simulink model "Target_Control_System"  (R2021b)
settings: Solver=FixedStepDiscrete  StartTime=0.0  StopTime=5  RelTol=1e-3
PreLoadFcn:
  | RTWConfigurationCB('preloadfcn', bdroot);
PostLoadFcn:
  | load('configuration/data_struct.mat');
  | load('configuration/fluxMaps_propMotor.mat');
  | load('configuration/parameterInit_PROP.mat');
  | load('configuration/parameterInit_PUMP.mat');
  | load('configuration/parameterInit_PITCH.mat');
  | load('configuration/parameterInit_TILT.mat');
  | %load('configuration/base_workspace_signal_definition.mat');
  | %load('resolvedatastores_to_baseworkspace_for_faster_simulation.mat');
model workspace (MAT data in the model file):
  SIMULATION_OPTIONS : Simulink.Parameter (value not decoded)
  TARGET_CODE_GEN : Simulink.Parameter (value not decoded)
  TCS_SAMPLE_FREQ_HZ : Simulink.Parameter (value not decoded)
symbols that are objects in the model workspace (value not decoded): TARGET_CODE_GEN, TCS_SAMPLE_FREQ_HZ
undefined symbols (not defined in the file): A_DQ_REF_LPF_INIT__PITCH, A_DQ_REF_LPF_INIT__PROP, A_DQ_REF_LPF_INIT__PUMP, A_DQ_REF_LPF_INIT__TILT, A_OBSERVER_CONFIDENCE_INIT__PITCH, A_OBSERVER_CONFIDENCE_INIT__PROP, A_OBSERVER_CONFIDENCE_INIT__PUMP, A_OBSERVER_CONFIDENCE_INIT__TILT, ACTUATOR_MAX_ANGLE_TRIP__PITCH, ACTUATOR_MIN_ANGLE_TRIP__PITCH, ACTUATOR_POS_SENSOR_INV_DIRECTION__PITCH, ACTUATOR_POS_SENSOR_INV_DIRECTION__TILT, ACTUATOR_POS_SENSOR_OFFSET__PITCH, ACTUATOR_POS_SENSOR_OFFSET__TILT, ADC_scaler1_baseaddr_TILT, ADC_SCALER_FLOAT_TO_FIXPOINT_EXPANSION, ANGLE_ELEC_FROM_SENSOR_OFFSET_INIT__PITCH, ANGLE_ELEC_FROM_SENSOR_OFFSET_INIT__PROP, ANGLE_ELEC_FROM_SENSOR_OFFSET_INIT__PUMP, ANGLE_ELEC_FROM_SENSOR_OFFSET_INIT__TILT, AUTO_CLEAR_FAULTS_ENABLED__PITCH, AUTO_CLEAR_FAULTS_ENABLED__PROP, AUTO_CLEAR_FAULTS_ENABLED__PUMP, AUTO_CLEAR_FAULTS_ENABLED__TILT, AUTO_CLEAR_FAULTS_WAIT_TICKS__PITCH, AUTO_CLEAR_FAULTS_WAIT_TICKS__PROP, AUTO_CLEAR_FAULTS_WAIT_TICKS__PUMP, AUTO_CLEAR_FAULTS_WAIT_TICKS__TILT, AUTO_I_ZERO_IDLE_TICKS__PITCH, AUTO_I_ZERO_IDLE_TICKS__PROP, AUTO_I_ZERO_IDLE_TICKS__PUMP, AUTO_I_ZERO_IDLE_TICKS__TILT, AUTO_I_ZERO_OFFSET_IDC_THRESHOLD__PITCH, AUTO_I_ZERO_OFFSET_IDC_THRESHOLD__PROP, AUTO_I_ZERO_OFFSET_IDC_THRESHOLD__PUMP, AUTO_I_ZERO_OFFSET_IDC_THRESHOLD__TILT, AUTO_I_ZERO_OFFSET_IPH_THRESHOLD__PITCH, AUTO_I_ZERO_OFFSET_IPH_THRESHOLD__PROP, AUTO_I_ZERO_OFFSET_IPH_THRESHOLD__PUMP, AUTO_I_ZERO_OFFSET_IPH_THRESHOLD__TILT, AUTO_SENSORLESS_SWITCHOVER_DISABLE_OMEGA, AUTO_SENSORLESS_SWITCHOVER_ENABLE_OMEGA, AUTO_SENSORLESS_SWITCHOVER_MIN_CONFIDENCE, AUXILIARY_PROTECTION_UNIT_BASEADDR__TILT, blanking_max_error_omega_INIT_PITCH, blanking_max_error_omega_INIT_TILT, blanking_max_error_position_INIT_PITCH, blanking_max_error_position_INIT_TILT, BRUTE_START_I_Q_REF_RAMP_SPEED__PITCH, BRUTE_START_I_Q_REF_RAMP_SPEED__PROP, BRUTE_START_I_Q_REF_RAMP_SPEED__PUMP, BRUTE_START_I_Q_REF_RAMP_SPEED__TILT, CONTROL_LOOP_DT_INIT__PITCH, CONTROL_LOOP_DT_INIT__PROP, CONTROL_LOOP_DT_INIT__PUMP, CONTROL_LOOP_DT_INIT__TILT, CORRECTION_FILTER_SCALE__PITCH, CORRECTION_FILTER_SCALE__PROP, CORRECTION_FILTER_SCALE__PUMP, CORRECTION_FILTER_SCALE__TILT ... (+458)
libraries: simulink x178, Reusables_Lib x24
(part 28 of 47)

== system Target_Control_System/Target_Control_System/MainLoop/pitchMotor_mainLoop/mainTask_pitch/motorTaskMainFastStep()/Lowpass Filtered Quantities for External World - Pitch ==
  lpfQuantities : TriggerPort  TriggerType=function-call  VariantControl=Variant
  Constant2 : Constant  Value=0.00008  OutDataTypeStr=single  SampleTime=-1
  Data Store Read27 : DataStoreRead  DataStoreName=oPitch  DataStoreElements=oPitch.oMot_.oParam_.fSlowPassFactor_  IndexOptions=Index vector (dialog)  Indices=1  OutputSizes=1
  Data Store Read28 : DataStoreRead  DataStoreName=oPitch  DataStoreElements=oPitch.oMot_.oIn_.fIPhaseMagnitude_  IndexOptions=Index vector (dialog)  Indices=1  OutputSizes=1
  Data Store Read29 : DataStoreRead  DataStoreName=oPitch  DataStoreElements=oPitch.oMot_.oState_.fIPhaseMagnitudeLpf_  IndexOptions=Index vector (dialog)  Indices=1  OutputSizes=1
  Data Store Read37 : DataStoreRead  DataStoreName=oPitch  DataStoreElements=oPitch.oMot_.oIn_.fId_  IndexOptions=Index vector (dialog)  Indices=1  OutputSizes=1
  Data Store Read42 : DataStoreRead  DataStoreName=oPitch  DataStoreElements=oPitch.oMot_.oIn_.fIq_  IndexOptions=Index vector (dialog)  Indices=1  OutputSizes=1
  Data Store Read43 : DataStoreRead  DataStoreName=oPitch  DataStoreElements=oPitch.oMot_.oOut_.fIdLpf_  IndexOptions=Index vector (dialog)  Indices=1  OutputSizes=1
  Data Store Read44 : DataStoreRead  DataStoreName=oPitch  DataStoreElements=oPitch.oMot_.oOut_.fIqLpf_  IndexOptions=Index vector (dialog)  Indices=1  OutputSizes=1
  Data Store Read46 : DataStoreRead  DataStoreName=oPitch  DataStoreElements=oPitch.oMot_.oOut_.fUdcLpf_  IndexOptions=Index vector (dialog)  Indices=1  OutputSizes=1
  Data Store Read47 : DataStoreRead  DataStoreName=oPitch  DataStoreElements=oPitch.oMot_.oIn_.oAdcData_.fIdc_  IndexOptions=Index vector (dialog)  Indices=1  OutputSizes=1
  Data Store Read48 : DataStoreRead  DataStoreName=oPitch  DataStoreElements=oPitch.oMot_.oOut_.fIdcLpf_  IndexOptions=Index vector (dialog)  Indices=1  OutputSizes=1
  Data Store Read49 : DataStoreRead  DataStoreName=oPitch  DataStoreElements=oPitch.oMot_.oIn_.fPowerDc_  IndexOptions=Index vector (dialog)  Indices=1  OutputSizes=1
  Data Store Read50 : DataStoreRead  DataStoreName=oPitch  DataStoreElements=oPitch.oMot_.oOut_.fPowerDcLpf_  IndexOptions=Index vector (dialog)  Indices=1  OutputSizes=1
  Data Store Read51 : DataStoreRead  DataStoreName=oPitch  DataStoreElements=oPitch.oMot_.oIn_.fTEstimate_  IndexOptions=Index vector (dialog)  Indices=1  OutputSizes=1
  Data Store Read52 : DataStoreRead  DataStoreName=oPitch  DataStoreElements=oPitch.oMot_.oOut_.fTEstimateLpf_  IndexOptions=Index vector (dialog)  Indices=1  OutputSizes=1
  Data Store Read53 : DataStoreRead  DataStoreName=oPitch  DataStoreElements=oPitch.oMot_.oState_.oRampDataIqRef_.fRampOut_  IndexOptions=Index vector (dialog)  Indices=1  OutputSizes=1
  Data Store Read54 : DataStoreRead  DataStoreName=oPitch  DataStoreElements=oPitch.oMot_.oOut_.fIqRefRampOutLpf_  IndexOptions=Index vector (dialog)  Indices=1  OutputSizes=1
  Data Store Read55 : DataStoreRead  DataStoreName=oPitch  DataStoreElements=oPitch.oMot_.oParam_.fADqRefLpf_  IndexOptions=Index vector (dialog)  Indices=1  OutputSizes=1
  Data Store Read56 : DataStoreRead  DataStoreName=oPitch  DataStoreElements=oPitch.oMot_.oIn_.fIdRefTotal_  IndexOptions=Index vector (dialog)  Indices=1  OutputSizes=1
  Data Store Read57 : DataStoreRead  DataStoreName=oPitch  DataStoreElements=oPitch.oMot_.oOut_.fIdRefLpf_  IndexOptions=Index vector (dialog)  Indices=1  OutputSizes=1
  Data Store Read58 : DataStoreRead  DataStoreName=oPitch  DataStoreElements=oPitch.oMot_.oIn_.fUqRef_  IndexOptions=Index vector (dialog)  Indices=1  OutputSizes=1
  Data Store Read59 : DataStoreRead  DataStoreName=oPitch  DataStoreElements=oPitch.oMot_.oOut_.fUqRefLpf_  IndexOptions=Index vector (dialog)  Indices=1  OutputSizes=1
  Data Store Read60 : DataStoreRead  DataStoreName=oPitch  DataStoreElements=oPitch.oMot_.oIn_.fUdRef_  IndexOptions=Index vector (dialog)  Indices=1  OutputSizes=1
  Data Store Read62 : DataStoreRead  DataStoreName=oPitch  DataStoreElements=oPitch.oMot_.oOut_.fUdRefLpf_  IndexOptions=Index vector (dialog)  Indices=1  OutputSizes=1
  Data Store Read63 : DataStoreRead  DataStoreName=oPitch  DataStoreElements=oPitch.oMot_.oOut_.fPowerDcLpf_  IndexOptions=Index vector (dialog)  Indices=1  OutputSizes=1
  Data Store Read64 : DataStoreRead  DataStoreName=oPitch  DataStoreElements=oPitch.oMot_.oOut_.fPowerDcXlpf_  IndexOptions=Index vector (dialog)  Indices=1  OutputSizes=1
  Data Store Read65 : DataStoreRead  DataStoreName=oPitch  DataStoreElements=oPitch.oMot_.oIn_.fOmegaEObserverLpf2_  IndexOptions=Index vector (dialog)  Indices=1  OutputSizes=1
  Data Store Read66 : DataStoreRead  DataStoreName=oPitch  DataStoreElements=oPitch.oMot_.oOut_.fOmegaEObserverXlpf2_  IndexOptions=Index vector (dialog)  Indices=1  OutputSizes=1
  Data Store Read69 : DataStoreRead  DataStoreName=oPitch  DataStoreElements=oPitch.oMot_.oParam_.fAOmegaXfilter2_  IndexOptions=Index vector (dialog)  Indices=1  OutputSizes=1
  Data Store Read77 : DataStoreRead  DataStoreName=oPitch  DataStoreElements=oPitch.oMot_.oIn_.oAdcData_.fUdc_  IndexOptions=Index vector (dialog)  Indices=1  OutputSizes=1
  Data Store Write20 : DataStoreWrite  DataStoreName=oPitch  DataStoreElements=oPitch.oMot_.oState_.fIPhaseMagnitudeLpf_  IndexOptions=Index vector (dialog)  Indices=1  OutputSizes=1
  Data Store Write21 : DataStoreWrite  DataStoreName=oPitch  DataStoreElements=oPitch.oMot_.oOut_.fIdLpf_  IndexOptions=Index vector (dialog)  Indices=1  OutputSizes=1
  Data Store Write22 : DataStoreWrite  DataStoreName=oPitch  DataStoreElements=oPitch.oMot_.oOut_.fIqLpf_  IndexOptions=Index vector (dialog)  Indices=1  OutputSizes=1
  Data Store Write24 : DataStoreWrite  DataStoreName=oPitch  DataStoreElements=oPitch.oMot_.oOut_.fUdcLpf_  IndexOptions=Index vector (dialog)  Indices=1  OutputSizes=1
  Data Store Write25 : DataStoreWrite  DataStoreName=oPitch  DataStoreElements=oPitch.oMot_.oOut_.fIdcLpf_  IndexOptions=Index vector (dialog)  Indices=1  OutputSizes=1
  Data Store Write28 : DataStoreWrite  DataStoreName=oPitch  DataStoreElements=oPitch.oMot_.oOut_.fPowerDcLpf_  IndexOptions=Index vector (dialog)  Indices=1  OutputSizes=1
  Data Store Write29 : DataStoreWrite  DataStoreName=oPitch  DataStoreElements=oPitch.oMot_.oOut_.fTEstimateLpf_  IndexOptions=Index vector (dialog)  Indices=1  OutputSizes=1
  Data Store Write30 : DataStoreWrite  DataStoreName=oPitch  DataStoreElements=oPitch.oMot_.oOut_.fIqRefRampOutLpf_  IndexOptions=Index vector (dialog)  Indices=1  OutputSizes=1
  Data Store Write31 : DataStoreWrite  DataStoreName=oPitch  DataStoreElements=oPitch.oMot_.oOut_.fIdRefLpf_  IndexOptions=Index vector (dialog)  Indices=1  OutputSizes=1
  Data Store Write32 : DataStoreWrite  DataStoreName=oPitch  DataStoreElements=oPitch.oMot_.oOut_.fUqRefLpf_  IndexOptions=Index vector (dialog)  Indices=1  OutputSizes=1
  Data Store Write34 : DataStoreWrite  DataStoreName=oPitch  DataStoreElements=oPitch.oMot_.oOut_.fUdRefLpf_  IndexOptions=Index vector (dialog)  Indices=1  OutputSizes=1
  Data Store Write35 : DataStoreWrite  DataStoreName=oPitch  DataStoreElements=oPitch.oMot_.oOut_.fPowerDcXlpf_  IndexOptions=Index vector (dialog)  Indices=1  OutputSizes=1
  Data Store Write36 : DataStoreWrite  DataStoreName=oPitch  DataStoreElements=oPitch.oMot_.oOut_.fOmegaEObserverXlpf2_  IndexOptions=Index vector (dialog)  Indices=1  OutputSizes=1
  Divide{8..20} (13 alike) : Product  Inputs=**
  Sum{4..5,7,10..11,13,15,18,20..22,25,29} (13 alike) : Sum  Inputs=|+-
  Sum{3,6,8..9,12,14,16..17,19,24,26,30..31} (13 alike) : Sum  Inputs=|++
  wires:
  Data Store Read27/1 -> Divide8/1, Divide9/1, Divide10/1, Divide12/1, Divide13/1, Divide14/1, Divide11/1
  Constant2/1 -> Divide20/1
  Sum12/1 -> Data Store Write25/1
  Sum6/1 -> Data Store Write21/1
  Sum8/1 -> Data Store Write22/1
  Data Store Read49/1 -> Sum11/1
  Data Store Read29/1 -> Sum7/2, Sum3/2
  Sum24/1 -> Data Store Write35/1
  Data Store Read47/1 -> Sum10/1
  Divide17/1 -> Sum30/1
  Sum3/1 -> Data Store Write20/1
  Data Store Read64/1 -> Sum24/2, Sum21/2
  Data Store Read54/1 -> Sum18/2, Sum17/2
  Divide13/1 -> Sum12/1
  Divide11/1 -> Sum14/1
  Divide16/1 -> Sum19/1
  Sum22/1 -> Divide18/2
  Sum15/1 -> Divide14/2
  Sum29/1 -> Divide17/2
  Sum4/1 -> Divide9/2
  Data Store Read58/1 -> Sum29/1
  Divide18/1 -> Sum26/1
  Sum21/1 -> Divide20/2
  Data Store Read42/1 -> Sum5/1
  Data Store Read77/1 -> Sum13/1
  Data Store Read59/1 -> Sum29/2, Sum30/2
  Divide20/1 -> Sum24/1
  Data Store Read69/1 -> Divide18/1
  Sum5/1 -> Divide10/2
  Sum31/1 -> Data Store Write34/1
  Sum16/1 -> Data Store Write29/1
  Sum19/1 -> Data Store Write31/1
  Sum7/1 -> Divide8/2
  Divide10/1 -> Sum8/1
  Data Store Read56/1 -> Sum20/1
  Sum18/1 -> Divide15/2
  Data Store Read28/1 -> Sum7/1
  Sum26/1 -> Data Store Write36/1
  Sum13/1 -> Divide12/2
  Data Store Read55/1 -> Divide15/1, Divide16/1, Divide19/1, Divide17/1
  Data Store Read57/1 -> Sum20/2, Sum19/2
  Divide8/1 -> Sum3/1
  Data Store Read65/1 -> Sum22/1
  Divide9/1 -> Sum6/1
  Data Store Read48/1 -> Sum12/2, Sum10/2
  Divide15/1 -> Sum17/1
  Data Store Read63/1 -> Sum21/1
  Divide14/1 -> Sum16/1
  Data Store Read43/1 -> Sum4/2, Sum6/2
  Data Store Read66/1 -> Sum26/2, Sum22/2
  Data Store Read53/1 -> Sum18/1
  Data Store Read44/1 -> Sum5/2, Sum8/2
  Data Store Read50/1 -> Sum14/2, Sum11/2
  Data Store Read52/1 -> Sum16/2, Sum15/2
  Sum30/1 -> Data Store Write32/1
  Sum17/1 -> Data Store Write30/1
  Data Store Read46/1 -> Sum9/2, Sum13/2
  Data Store Read37/1 -> Sum4/1
  Sum11/1 -> Divide11/2
  Divide12/1 -> Sum9/1
  Data Store Read60/1 -> Sum25/1
  Sum10/1 -> Divide13/2
  Divide19/1 -> Sum31/1
  Sum25/1 -> Divide19/2
  Data Store Read62/1 -> Sum25/2, Sum31/2
  Data Store Read51/1 -> Sum15/1
  Sum14/1 -> Data Store Write28/1
  Sum9/1 -> Data Store Write24/1
  Sum20/1 -> Divide16/2

== system Target_Control_System/Target_Control_System/MainLoop/pitchMotor_mainLoop/mainTask_pitch/motorTaskMainFastStep()/Mechanical System - Pitch ==
  mechanicalSystem : TriggerPort  TriggerType=function-call  VariantControl=Variant
  Data Store Read : DataStoreRead  DataStoreName=oPitch  DataStoreElements=oPitch.oMot_.oState_.oPosSensor_.eInputPositionSensorType_  IndexOptions=Index vector (dialog)  Indices=1  OutputSizes=1
  Enumerated Constant1 : simulink/Sources/Enumerated Constant  OutDataTypeStr=Enum: EPositionSensor_t  Value=EPositionSensor_t.eNone  SampleTime=-1
  NotEqual : RelationalOperator  Operator=~=  OutDataTypeStr=boolean  RndMeth=Simplest
  processSensors(&oPitch) : Subsystem  TreatAsAtomicUnit=on
  wires:
  Enumerated Constant1/1 -> NotEqual/2
  NotEqual/1 -> processSensors(&oPitch)/Enable
  Data Store Read/1 -> NotEqual/1

== system Target_Control_System/Target_Control_System/MainLoop/pitchMotor_mainLoop/mainTask_pitch/motorTaskMainFastStep()/Motor Acceleration - Pitch ==
  note: // Compute the acceleration (derivative of the speed). It is computed simply from the 1-step difference,
      |    // but strongly low pass filtered to ultimately end up with a bandwidth less than 50-100 Hz.
      |    // A filter running at the typical control frequency (80 kHz for the prop) would have to be too steep, so
      |    // a multi-stage, dual sample rate approach is used: A first filter runs at full control rate, with a cut-
      |    // off frequency of some 1-2 kHz. A second filter runs at 5 kHz and brings the bandwidth down to less than
      |    // 50-100 Hz.
      |    // At this location in the code, the first filter stage is executed:
  motorAcceleration : TriggerPort  TriggerType=function-call  VariantControl=Variant
  First filter stage : Subsystem  TreatAsAtomicUnit=on
  Function-Call Generator : simulink/Ports & Subsystems/Function-Call Generator  sample_time=-1  numberOfIterations=1  DisallowWideOutput=off
  Function-Call Split10 : FunctionCallSplit  NumOutputPorts=2
  Speed step : Subsystem
  wires:
  Function-Call Generator/1 -> Function-Call Split10/1
  Function-Call Split10/1 -> First filter stage/Trigger
  Function-Call Split10/2 -> Speed step/Trigger

== system Target_Control_System/Target_Control_System/MainLoop/pitchMotor_mainLoop/mainTask_pitch/motorTaskMainFastStep()/Observer Confidence - Pitch ==
  note: // ideally zero,
      | // but can go up to inf
  note: // Three contributions, each adding 1/3 to give a value in range 0.0-1.0:
      | //  1. Magnitude of estimated flux relative to nominal flux (perhaps not for induction motors)
      | //  REMOVED (for the time being) 2. The relative noise on the magnitude of the estimated flux (relative noise=magnitude of derivative/HPF divided by average value)
      | //  3. The relative noise on the estimated speed
  note: // If greater than 125% off,
      | // keep at 125%
  note: // the 0.4 is 0.5/tempf_max
  note: // 1. magnitude of flux. Map to a 0-0.33 range
  note: // 3. noise on estimated omega
  note: // ideally zero,
      | // but can go up to inf
  note: // If greater than X% off,
      | // keep at X%
  observerConfidence : TriggerPort  TriggerType=function-call  VariantControl=Variant
  Abs2 : Abs  OutDataTypeStr=single
  Abs3 : Abs  OutDataTypeStr=single
  Abs5 : Abs  OutDataTypeStr=single
  Add10 : Sum  Inputs=|-+
  Add11 : Sum
  Add2 : Sum  Inputs=+-
  Add7 : Sum  Inputs=|+-
  Add8 : Sum  Inputs=|-+
  Add9 : Sum  Inputs=|-+
  Automatic switching to sensorless : Subsystem  TreatAsAtomicUnit=on
  Constant14 : Constant  OutDataTypeStr=single  SampleTime=-1
  Data Store Read1 : DataStoreRead  DataStoreName=oPitch  DataStoreElements=oPitch.oMot_.oParam_.fAObserverConfidence_  IndexOptions=Index vector (dialog)  Indices=1  OutputSizes=1
  Data Store Read11 : DataStoreRead  DataStoreName=oPitch  DataStoreElements=oPitch.oMot_.oOut_.fOmegaEObserverXlpf2_  IndexOptions=Index vector (dialog)  Indices=1  OutputSizes=1
  Data Store Read13 : DataStoreRead  DataStoreName=oPitch  DataStoreElements=oPitch.oMot_.oIn_.fFluxMainMagnitudeLpf_  IndexOptions=Index vector (dialog)  Indices=1  OutputSizes=1
  Data Store Read4 : DataStoreRead  DataStoreName=oPitch  DataStoreElements=oPitch.oMot_.oParam_.uiSensorlessSwitchoverMode_  IndexOptions=Index vector (dialog)  Indices=1  OutputSizes=1
  Data Store Read61 : DataStoreRead  DataStoreName=oPitch  DataStoreElements=oPitch.oIsr_.oState_.fOmegaEObserverRaw2_  IndexOptions=Index vector (dialog)  Indices=1  OutputSizes=1
  Data Store Read83 : DataStoreRead  DataStoreName=oPitch  DataStoreElements=oPitch.oMot_.oParam_.fMainFluxNominal_  IndexOptions=Index vector (dialog)  Indices=1  OutputSizes=1
  Data Store Write33 : DataStoreWrite  DataStoreName=oPitch  DataStoreElements=oPitch.oMot_.oState_.fObserverConfidence_  IndexOptions=Index vector (dialog)  Indices=1  OutputSizes=1
  Divide1 : Product  Inputs=*/
  Divide3 : Product  Inputs=*/
  Gain11 : Gain  Gain=0.83
  Gain5 : Gain  Gain=0.4
  Half : Constant  Value=0.5  OutDataTypeStr=single  SampleTime=-1
  Half2 : Constant  Value=0.5  OutDataTypeStr=single  SampleTime=-1
  IIR : Subsystem
  Saturation2 : Saturate  UpperLimit=1.25  LowerLimit=-inf
  Saturation3 : Saturate  UpperLimit=0.6  LowerLimit=-inf
  Switch3 : Switch  Criteria=u2 > Threshold  Threshold=0.5
  Zero8 : Constant  Value=0  OutDataTypeStr=Inherit: Inherit via back propagation  SampleTime=-1
  isNaN : RelationalOperator  Operator=isNaN  OutDataTypeStr=boolean  RndMeth=Simplest
  wires:
  Zero8/1 -> Switch3/1
  Half2/1 -> Add10/2
  Data Store Read13/1 -> Add7/1
  Data Store Read4/1 -> Automatic switching to sensorless/Enable
  Half/1 -> Add8/2
  Switch3/1 -> IIR/1(In)  "fObserverConfidenceRaw"
  Divide3/1 -> Saturation3/1
  Data Store Read83/1 -> Add7/2, Divide1/2
  Data Store Read11/1 -> Abs5/1, Add9/2
  Add10/1 -> Add11/2
  Abs5/1 -> Divide3/2
  Constant14/1 -> Add2/1
  Add8/1 -> Add11/1
  Data Store Read1/1 -> IIR/3(K), Add2/2
  Saturation2/1 -> Gain5/1  "fTemp"
  Divide1/1 -> Saturation2/1
  Add7/1 -> Abs2/1
  Gain11/1 -> Add10/1
  IIR/1(Out) -> Automatic switching to sensorless/1(In1), Data Store Write33/1
  Add11/1 -> Switch3/3, isNaN/1  "fObserverConfidenceRaw"
  Add9/1 -> Abs3/1
  Add2/1 -> IIR/2(1-K)
  Abs3/1 -> Divide3/1
  Abs2/1 -> Divide1/1
  isNaN/1 -> Switch3/2
  Saturation3/1 -> Gain11/1
  Data Store Read61/1 -> Add9/1
  Gain5/1 -> Add8/1

== system Target_Control_System/Target_Control_System/MainLoop/pitchMotor_mainLoop/mainTask_pitch/motorTaskMainFastStep()/Software Overcurrent Protection - Pitch ==
  overcurrentProtection : TriggerPort  TriggerType=function-call  VariantControl=Variant
  Constant7 : Constant  Value=211  OutDataTypeStr=uint32  SampleTime=-1
  Constant8 : Constant  Value=212  OutDataTypeStr=uint32  SampleTime=-1
  Data Store Read45 : DataStoreRead  DataStoreName=oPitch  DataStoreElements=oPitch.oMot_.oIn_.fIPhaseMagnitude_  IndexOptions=Index vector (dialog)  Indices=1  OutputSizes=1
  Data Store Read79 : DataStoreRead  DataStoreName=oPitch  DataStoreElements=oPitch.oMot_.oState_.uiDriveState_  IndexOptions=Index vector (dialog)  Indices=1  OutputSizes=1
  Data Store Read81 : DataStoreRead  DataStoreName=oPitch  DataStoreElements=oPitch.oMot_.oParam_.fTripLimitSoftwareA_  IndexOptions=Index vector (dialog)  Indices=1  OutputSizes=1
  Equal1 : RelationalOperator  Operator===  OutDataTypeStr=boolean  RndMeth=Simplest
  Equal2 : RelationalOperator  Operator===  OutDataTypeStr=boolean  RndMeth=Simplest
  Forced_angle_overcurrent : Subsystem  TreatAsAtomicUnit=on
  GreaterThan3 : RelationalOperator  Operator=>  OutDataTypeStr=boolean  RndMeth=Simplest
  OR : Logic  Operator=OR  AllPortsSameDT=off  OutDataTypeStr=boolean
  checkForHwOvercurrents(&oPitch) : Subsystem  TreatAsAtomicUnit=on
  softwareOvercurrentProtection : Stateflow chart  TreatAsAtomicUnit=on
  wires:
  Constant8/1 -> Equal2/1
  Equal2/1 -> OR/1
  Equal1/1 -> OR/2
  OR/1 -> Forced_angle_overcurrent/Enable
  Data Store Read79/1 -> Equal1/1, Equal2/2
  Constant7/1 -> Equal1/2
  GreaterThan3/1 -> checkForHwOvercurrents(&oPitch)/Enable
  Data Store Read45/1 -> GreaterThan3/1
  Data Store Read81/1 -> GreaterThan3/2

== system Target_Control_System/Target_Control_System/MainLoop/propMotor_mainLoop/Decimation gate A for 200 Hz Prop/Current offset nulling/initiateOffsetNulling(&oProp) ==
  note: Further checks for starting the nulling process are handled inside the lower level function
  Enable : EnablePort
  Chart : Stateflow chart  TreatAsAtomicUnit=on

== system Target_Control_System/Target_Control_System/MainLoop/propMotor_mainLoop/Decimation gate A for 200 Hz Prop/Subsystem/Subsystem ==
  Enable : EnablePort
  Data Store Write1 : DataStoreWrite  DataStoreName=oProp  DataStoreElements=oProp.oMot_.oState_.fIdleCtrlCurrent_  IndexOptions=Index vector (dialog)  Indices=1  OutputSizes=1
  Data Store Write3 : DataStoreWrite  DataStoreName=oProp  DataStoreElements=oProp.oMot_.oParam_.oPiDataIdleCtrl_.fState_  IndexOptions=Index vector (dialog)  Indices=1  OutputSizes=1
  Zero1 : Constant  Value=0  OutDataTypeStr=single  SampleTime=-1
  wires:
  Zero1/1 -> Data Store Write1/1, Data Store Write3/1

== system Target_Control_System/Target_Control_System/MainLoop/propMotor_mainLoop/Decimation gate A for 200 Hz Prop/Subsystem/piControllerStep_Idle_Controller ==
  fActual : Inport
  fTarget : Inport  Port=2
  fKp : Inport  Port=3
  fKi : Inport  Port=4
  fScale : Inport  Port=5
  fLoopDt : Inport  Port=6
  fIntMax : Inport  Port=7
  fOutMax : Inport  Port=8
  fIntMin : Inport  Port=9
  fOutMin : Inport  Port=10
  fState : Inport  Port=11
  Enable : EnablePort
  Add : Sum  Inputs=|++
  Data Store Write11 : DataStoreWrite  DataStoreName=oProp  DataStoreElements=oProp.oMot_.oState_.fIdleCtrlCurrent_  IndexOptions=Index vector (dialog)  Indices=1  OutputSizes=1
  Data Store Write2 : DataStoreWrite  DataStoreName=oProp  DataStoreElements=oProp.oMot_.oParam_.oPiDataIdleCtrl_.fState_  IndexOptions=Index vector (dialog)  Indices=1  OutputSizes=1
  Mux : Mux  Inputs=3
  Mux1 : Mux  Inputs=3
  Product : Product
  Saturation Dynamic : simulink/Discontinuities/Saturation Dynamic  OutMin=[]  OutMax=[]  OutDataTypeStr=Inherit: Same as second input  OutDataType=fixdt(1, 16)  OutScaling=2^-10  DoSatur=off
  Saturation Dynamic1 : simulink/Discontinuities/Saturation Dynamic  OutMin=[]  OutMax=[]  OutDataTypeStr=Inherit: Same as second input  OutDataType=fixdt(1, 16)  OutScaling=2^-10  DoSatur=off
  Scope3 : Scope  NumInputPorts=6
  Sum1 : Sum  Inputs=++|
  Sum22 : Sum  Inputs=-+|
  fError * fKi_ * fScale : Fcn  Expr=u(1)*u(2)*u(3)
  fError * fKp_ * fScale1 : Fcn  Expr=u(1)*u(2)*u(3)
  wires:
  Saturation Dynamic1/1 -> Scope3/6, Data Store Write11/1  "fIdleCtrlCurrent_"
  fLoopDt/1 -> Product/2
  fOutMax/1 -> Saturation Dynamic1/1
  fOutMin/1 -> Saturation Dynamic1/3
  fIntMin/1 -> Saturation Dynamic/3
  fIntMax/1 -> Saturation Dynamic/1
  Add/1 -> Saturation Dynamic/2
  fState/1 -> Add/2
  Product/1 -> Add/1
  Mux1/1 -> fError * fKp_ * fScale1/1
  fKi/1 -> Mux/2
  fScale/1 -> Mux/1, Mux1/3
  fKp/1 -> Mux1/2
  Mux/1 -> fError * fKi_ * fScale/1
  Sum1/1 -> Saturation Dynamic1/2  "fError"
  fError * fKp_ * fScale1/1 -> Sum1/1, Scope3/4
  Saturation Dynamic/1 -> Scope3/5, Data Store Write2/1, Sum1/2  "*fpState"
  fActual/1 -> Sum22/1, Scope3/2
  fTarget/1 -> Sum22/2, Scope3/1
  fError * fKi_ * fScale/1 -> Product/1
  Sum22/1 -> Scope3/3, Mux/3, Mux1/1  "fError"

== system Target_Control_System/Target_Control_System/MainLoop/propMotor_mainLoop/Decimation gate for 5000 Hz Prop/motorTaskProcessExternalSetpoints(&oProp)/Subsystem1 ==
  passive_holding_mode : TriggerPort  TriggerType=function-call  VariantControl=Variant
  AND5 : Logic  Operator=OR  Inputs=3  AllPortsSameDT=off  OutDataTypeStr=boolean
  Data Store Read85 : DataStoreRead  DataStoreName=oProp  DataStoreElements=oProp.oMot_.oState_.uiDriveState_  IndexOptions=Index vector (dialog)  Indices=1  OutputSizes=1
  Equal1 : RelationalOperator  Operator===  OutDataTypeStr=boolean  RndMeth=Simplest
  Equal13 : RelationalOperator  Operator===  OutDataTypeStr=boolean  RndMeth=Simplest
  Equal2 : RelationalOperator  Operator===  OutDataTypeStr=boolean  RndMeth=Simplest
  Subsystem : Subsystem
  const1 : Constant  Value=226  OutDataTypeStr=uint32  SampleTime=-1
  const2 : Constant  Value=227  OutDataTypeStr=uint32  SampleTime=-1
  const3 : Constant  Value=228  OutDataTypeStr=uint32  SampleTime=-1
  wires:
  const3/1 -> Equal2/2
  const2/1 -> Equal1/2
  const1/1 -> Equal13/2
  Data Store Read85/1 -> Equal13/1, Equal1/1, Equal2/1
  Equal1/1 -> AND5/2
  Equal2/1 -> AND5/3
  AND5/1 -> Subsystem/Enable
  Equal13/1 -> AND5/1

== system Target_Control_System/Target_Control_System/MainLoop/propMotor_mainLoop/Decimation gate for 5000 Hz Prop/motorTaskProcessExternalSetpoints(&oProp)/Subsystem2 ==
  hot_standby : TriggerPort  TriggerType=function-call  VariantControl=Variant
  AND5 : Logic  Operator=OR  AllPortsSameDT=off  OutDataTypeStr=boolean
  Data Store Read85 : DataStoreRead  DataStoreName=oProp  DataStoreElements=oProp.oMot_.oState_.uiDriveState_  IndexOptions=Index vector (dialog)  Indices=1  OutputSizes=1
  Equal1 : RelationalOperator  Operator===  OutDataTypeStr=boolean  RndMeth=Simplest
  Equal13 : RelationalOperator  Operator===  OutDataTypeStr=boolean  RndMeth=Simplest
  Subsystem : Subsystem
  const1 : Constant  Value=235  OutDataTypeStr=uint32  SampleTime=-1
  const2 : Constant  Value=236  OutDataTypeStr=uint32  SampleTime=-1
  wires:
  const2/1 -> Equal1/2
  const1/1 -> Equal13/2
  Data Store Read85/1 -> Equal13/1, Equal1/1
  Equal1/1 -> AND5/2
  AND5/1 -> Subsystem/Enable
  Equal13/1 -> AND5/1

== system Target_Control_System/Target_Control_System/MainLoop/propMotor_mainLoop/Decimation gate for 5000 Hz Prop/motorTaskProcessExternalSetpoints(&oProp)/Subsystem3 ==
  note: // Position target
  note: // Speed target
  note: Iq current (that is, torque target)
  note: // Do Id
  note: // (Iq is controlled by the forced angle sequencer)
  note: // Forced angle start regime, ensure that Id is zero
  set_target : TriggerPort  TriggerType=function-call  VariantControl=Variant
  AND1 : Logic  AllPortsSameDT=off  OutDataTypeStr=boolean
  AND5 : Logic  Inputs=3  AllPortsSameDT=off  OutDataTypeStr=boolean
  Data Store Read85 : DataStoreRead  DataStoreName=oProp  DataStoreElements=oProp.oMot_.oState_.uiDriveState_  IndexOptions=Index vector (dialog)  Indices=1  OutputSizes=1
  Equal1 : RelationalOperator  OutDataTypeStr=boolean  RndMeth=Simplest
  Equal13 : RelationalOperator  Operator=~=  OutDataTypeStr=boolean  RndMeth=Simplest
  Equal14 : RelationalOperator  Operator=~=  OutDataTypeStr=boolean  RndMeth=Simplest
  Equal2 : RelationalOperator  Operator=<=  OutDataTypeStr=boolean  RndMeth=Simplest
  NOT : Logic  Operator=NOT  AllPortsSameDT=off  OutDataTypeStr=boolean
  NOT1 : Logic  Operator=NOT  AllPortsSameDT=off  OutDataTypeStr=boolean
  Subsystem : Subsystem
  Subsystem1 : Subsystem
  Subsystem2 : Subsystem
  Subsystem3 : Subsystem
  Subsystem4 : Subsystem
  const1 : Constant  Value=245  OutDataTypeStr=uint32  SampleTime=-1
  const17 : Constant  Value=211  OutDataTypeStr=uint32  SampleTime=-1
  const18 : Constant  Value=212  OutDataTypeStr=uint32  SampleTime=-1
  const2 : Constant  Value=254  OutDataTypeStr=uint32  SampleTime=-1
  wires:
  NOT1/1 -> Subsystem4/Enable
  AND5/1 -> NOT1/1, Subsystem3/Enable, Subsystem/Enable, Subsystem1/Enable, Subsystem2/Enable
  Equal13/1 -> AND5/1
  Equal1/1 -> AND1/1
  const18/1 -> Equal14/2
  Equal2/1 -> AND1/2
  AND1/1 -> NOT/1
  const17/1 -> Equal13/1
  Data Store Read85/1 -> Equal2/1, Equal1/1, Equal14/1, Equal13/2
  const2/1 -> Equal2/2
  NOT/1 -> AND5/3
  const1/1 -> Equal1/2
  Equal14/1 -> AND5/2

== system Target_Control_System/Target_Control_System/MainLoop/propMotor_mainLoop/motorTaskMainFastStep(&oProp)/Control Loops - Prop/Dynamic Current Limiting Prop ==
  Enable : EnablePort
  Abs : Abs
  Add : Sum  Inputs=+-
  Add1 : Sum
  Add2 : Sum  Inputs=-+
  Data Store Read : DataStoreRead  DataStoreName=oProp  DataStoreElements=oProp.oMot_.oIn_.fIPhaseMagnitude_  IndexOptions=Index vector (dialog)  Indices=1  OutputSizes=1
  Data Store Read1 : DataStoreRead  DataStoreName=oProp  DataStoreElements=oProp.oMot_.oParam_.fIqSetpointMax_  IndexOptions=Index vector (dialog)  Indices=1  OutputSizes=1
  Data Store Read10 : DataStoreRead  DataStoreName=oProp  DataStoreElements=oProp.oMot_.oParam_.fDynILimIntegratorLeakageFactor_  IndexOptions=Index vector (dialog)  Indices=1  OutputSizes=1
  Data Store Read2 : DataStoreRead  DataStoreName=oProp  DataStoreElements=oProp.oMot_.oState_.fDynILimIntegrator_  IndexOptions=Index vector (dialog)  Indices=1  OutputSizes=1
  Data Store Read3 : DataStoreRead  DataStoreName=oProp  DataStoreElements=oProp.oMot_.oParam_.fDynILimDynamicMax_  IndexOptions=Index vector (dialog)  Indices=1  OutputSizes=1
  Data Store Read4 : DataStoreRead  DataStoreName=oProp  DataStoreElements=oProp.oMot_.oParam_.fTorqueAuthorityFraction_  IndexOptions=Index vector (dialog)  Indices=1  OutputSizes=1
  Data Store Read5 : DataStoreRead  DataStoreName=oProp  DataStoreElements=oProp.oMot_.oParam_.fDynILimKnockdownFactor_  IndexOptions=Index vector (dialog)  Indices=1  OutputSizes=1
  Data Store Read6 : DataStoreRead  DataStoreName=oProp  DataStoreElements=oProp.oMot_.oState_.fIqRefBeforeRamp_  IndexOptions=Index vector (dialog)  Indices=1  OutputSizes=1
  Data Store Read7 : DataStoreRead  DataStoreName=oProp  DataStoreElements=oProp.oMot_.oParam_.fDynILimDynamicMax_  IndexOptions=Index vector (dialog)  Indices=1  OutputSizes=1
  Data Store Write : DataStoreWrite  DataStoreName=oProp  DataStoreElements=oProp.oMot_.oState_.fDynILimIntegrator_  IndexOptions=Index vector (dialog)  Indices=1  OutputSizes=1
  Data Store Write1 : DataStoreWrite  DataStoreName=oProp  DataStoreElements=oProp.oMot_.oState_.fDynILimActualLimit_  IndexOptions=Index vector (dialog)  Indices=1  OutputSizes=1
  Data Store Write3 : DataStoreWrite  DataStoreName=oProp  DataStoreElements=oProp.oMot_.oParam_.oPid2DataRpmCtrl_.oParameter_.fOutMax_  IndexOptions=Index vector (dialog)  Indices=1  OutputSizes=1
  Data Store Write4 : DataStoreWrite  DataStoreName=oProp  DataStoreElements=oProp.oMot_.oParam_.oPid2DataRpmCtrl_.oParameter_.fOutMin_  IndexOptions=Index vector (dialog)  Indices=1  OutputSizes=1
  Data Store Write5 : DataStoreWrite  DataStoreName=oProp  DataStoreElements=oProp.oMot_.oParam_.oPid2DataRpmCtrl_.oParameter_.fIntMin_  IndexOptions=Index vector (dialog)  Indices=1  OutputSizes=1
  Data Store Write6 : DataStoreWrite  DataStoreName=oProp  DataStoreElements=oProp.oMot_.oParam_.oPid2DataRpmCtrl_.oParameter_.fIntMax_  IndexOptions=Index vector (dialog)  Indices=1  OutputSizes=1
  Divide{,1..3} (4 alike) : Product  Inputs=**
  Gain : Gain  Gain=-1
  Gain1 : Gain  Gain=-1
  Gain2 : Gain  Gain=-1
  Max : MinMax  Function=max  Inputs=2
  Max1 : MinMax  Function=max  Inputs=2
  Min : MinMax  Inputs=2
  Switch : Switch  Criteria=u2 > Threshold
  oRampDataIqRef_.fSetpoint : Outport
  wires:
  Gain2/1 -> Data Store Write4/1
  Data Store Read7/1 -> Gain2/1, Data Store Write3/1
  Gain1/1 -> Data Store Write5/1
  Max1/1 -> oRampDataIqRef_.fSetpoint/1
  Gain/1 -> Max1/1
  Min/1 -> Max1/2
  Data Store Read6/1 -> Min/2
  Max/1 -> Min/1, Data Store Write1/1, Gain1/1, Data Store Write6/1, Gain/1
  Add2/1 -> Max/1
  Divide2/1 -> Add2/2
  Divide3/1 -> Add2/1
  Data Store Read5/1 -> Divide3/2
  Data Store Read4/1 -> Divide2/2
  Data Store Read3/1 -> Divide2/1
  Divide1/1 -> Switch/3
  Data Store Read10/1 -> Divide1/2
  Data Store Read2/1 -> Add1/2, Divide1/1
  Divide/1 -> Add1/1
  Switch/1 -> Divide3/1, Data Store Write/1
  Add1/1 -> Switch/1
  Add/1 -> Switch/2, Divide/2, Divide/1  "fTemp"
  Abs/1 -> Add/1
  Data Store Read1/1 -> Add/2, Max/2
  Data Store Read/1 -> Abs/1

== system Target_Control_System/Target_Control_System/MainLoop/propMotor_mainLoop/motorTaskMainFastStep(&oProp)/Control Loops - Prop/Sim Options Prop Id Variant Subsystem ==
  note: 1) Add Subsystem or Model blocks as valid variant choices.
      | 2) You cannot connect blocks at this level. At simulation, connectivity is automatically
      | determined, based on the active variant and port name matching.
  Sim Options 0 Prop Id Subsystem : Subsystem  VariantControl=(default)
  Sim Options 1 Prop Iq Subsystem : Subsystem  VariantControl=SIMULATION_OPTIONS == 1 && TARGET_CODE_GEN ~= 1
  Out1 : Outport

== system Target_Control_System/Target_Control_System/MainLoop/propMotor_mainLoop/motorTaskMainFastStep(&oProp)/Control Loops - Prop/Sim Options Prop Iq Variant Subsystem ==
  note: 1) Add Subsystem or Model blocks as valid variant choices.
      | 2) You cannot connect blocks at this level. At simulation, connectivity is automatically
      | determined, based on the active variant and port name matching.
  Sim Options 0 Prop Iq Subsystem : Subsystem  VariantControl=(default)
  Sim Options 1 Prop Iq Subsystem : Subsystem  VariantControl=SIMULATION_OPTIONS == 1 && TARGET_CODE_GEN ~= 1
  Out1 : Outport

== system Target_Control_System/Target_Control_System/MainLoop/propMotor_mainLoop/motorTaskMainFastStep(&oProp)/Control Loops - Prop/Subsystem2 ==
  Enable : EnablePort
  Data Store Read2 : DataStoreRead  DataStoreName=oProp  DataStoreElements=oProp.oMot_.oIn_.fUdRef_  IndexOptions=Index vector (dialog)  Indices=1  OutputSizes=1
  Data Store Read3 : DataStoreRead  DataStoreName=oProp  DataStoreElements=oProp.oMot_.oIn_.fUqRef_  IndexOptions=Index vector (dialog)  Indices=1  OutputSizes=1
  Data Store Read5 : DataStoreRead  DataStoreName=oProp  DataStoreElements=oProp.oMot_.oState_.fFluxWeakeningState_  IndexOptions=Index vector (dialog)  Indices=1  OutputSizes=1
  Data Store Read6 : DataStoreRead  DataStoreName=oProp  DataStoreElements=oProp.oMot_.oParam_.fFluxWeakeningModulationTarget_  IndexOptions=Index vector (dialog)  Indices=1  OutputSizes=1
  Data Store Read69 : DataStoreRead  DataStoreName=oProp  DataStoreElements=oProp.oMot_.oParam_.fFluxWeakeningDownRamp_  IndexOptions=Index vector (dialog)  Indices=1  OutputSizes=1
  Data Store Read94 : DataStoreRead  DataStoreName=oProp  DataStoreElements=oProp.oMot_.oState_.fFluxWeakeningState_  IndexOptions=Index vector (dialog)  Indices=1  OutputSizes=1
  Data Store Read95 : DataStoreRead  DataStoreName=oProp  DataStoreElements=oProp.oMot_.oParam_.fIntControlLoopDt_  IndexOptions=Index vector (dialog)  Indices=1  OutputSizes=1
  Data Store Read96 : DataStoreRead  DataStoreName=oProp  DataStoreElements=oProp.oMot_.oParam_.fIntControlLoopDt_  IndexOptions=Index vector (dialog)  Indices=1  OutputSizes=1
  Equal13 : RelationalOperator  Operator=<  OutDataTypeStr=boolean  RndMeth=Simplest
  Mux : Mux  Inputs=2
  NOT1 : Logic  Operator=NOT  AllPortsSameDT=off  OutDataTypeStr=boolean
  Square Sum : Fcn  Expr=u(1)*u(1)+u(2)*u(2)
  Subsystem : Subsystem
  Subsystem1 : Subsystem
  Switch1 : Switch  Criteria=u2 > Threshold  Threshold=0.5
  Out1 : Outport
  wires:
  Subsystem1/1(Out1) -> Switch1/1
  NOT1/1 -> Subsystem/Enable
  Data Store Read94/1 -> Subsystem/3(fFluxWeakeningState_)
  Subsystem/1(Out1) -> Switch1/3
  Mux/1 -> Square Sum/1
  Data Store Read95/1 -> Subsystem/4(fIntControlLoopDt_)
  Data Store Read6/1 -> Equal13/2, Subsystem/1(fFluxWeakeningModulationTarget_)  "fFluxWeakeningModulationTarget_"
  Square Sum/1 -> Subsystem/2(fModulationIndexSquared), Equal13/1  "fModulationIndexSquared_"
  Data Store Read3/1 -> Mux/2
  Equal13/1 -> Subsystem1/Enable, NOT1/1, Switch1/2
  Data Store Read96/1 -> Subsystem1/2(fIntControlLoopDt_)
  Switch1/1 -> Out1/1
  Data Store Read2/1 -> Mux/1
  Data Store Read69/1 -> Subsystem1/1(fFluxWeakeningDownRamp_)
  Data Store Read5/1 -> Subsystem1/3(fFluxWeakeningState_)

== system Target_Control_System/Target_Control_System/MainLoop/propMotor_mainLoop/motorTaskMainFastStep(&oProp)/Control Loops - Prop/rampStep_oRampDataIqRef_ ==
  note: U(k)
  note: Y(k)
  fSetpoint_ : Inport
  fUpslope_ : Inport  Port=2
  fDDownslope_ : Inport  Port=3
  fTimestepS_ : Inport  Port=4
  fRampOut_z : Inport  Port=5
  Difference Inputs1 : Sum  Description=Add in CPU  DisableCoverage=on  Inputs=+-  OutDataTypeStr=Inherit: Inherit via back propagation
  Difference Inputs2 : Sum  Description=Add in CPU  OutDataTypeStr=Inherit: Inherit via back propagation
  Difference Inputs3 : Sum  Description=Add in CPU  DisableCoverage=on  Inputs=+-  OutDataTypeStr=Inherit: Inherit via back propagation
  Gain : Gain  Gain=-1
  Saturation Dynamic : simulink/Discontinuities/Saturation Dynamic  OutMin=[]  OutMax=[]  OutDataTypeStr=Inherit: Same as second input  OutDataType=fixdt(1, 16)  OutScaling=2^-10  DoSatur=off
  delta fall limit : Product  DisableCoverage=on  Inputs=**  OutDataTypeStr=Inherit: Inherit via back propagation  SaturateOnIntegerOverflow=on
  delta fall limit1 : Product  DisableCoverage=on  Inputs=*/  OutDataTypeStr=Inherit: Inherit via back propagation  SaturateOnIntegerOverflow=on
  delta rise limit : Product  DisableCoverage=on  Inputs=**  OutDataTypeStr=Inherit: Inherit via back propagation  SaturateOnIntegerOverflow=on
  fRampOut_ : Outport  InitialOutput=0
  fRampOutDdt_ : Outport  Port=2  InitialOutput=0
  wires:
  fRampOut_z/1 -> Difference Inputs1/2, Difference Inputs2/2, Difference Inputs3/2
  Difference Inputs1/1 -> Saturation Dynamic/2  "( U(k) - Y(k-1) )"
  fDDownslope_/1 -> Gain/1
  delta rise limit/1 -> Saturation Dynamic/1
  fSetpoint_/1 -> Difference Inputs1/1
  delta fall limit/1 -> Saturation Dynamic/3
  fUpslope_/1 -> delta rise limit/1
  Difference Inputs2/1 -> Difference Inputs3/1, fRampOut_/1
  Saturation Dynamic/1 -> Difference Inputs2/1
  fTimestepS_/1 -> delta fall limit1/2, delta fall limit/2, delta rise limit/2
  Difference Inputs3/1 -> delta fall limit1/1  "( Y(k) - Y(k-1) )"
  delta fall limit1/1 -> fRampOutDdt_/1
  Gain/1 -> delta fall limit/1

== system Target_Control_System/Target_Control_System/MainLoop/propMotor_mainLoop/motorTaskMainFastStep(&oProp)/Correction Constants for Observer and Control - Prop/Variant Subsystem ==
  note: 1) Add Subsystem or Model blocks as valid variant choices.
      | 2) You cannot connect blocks at this level. At simulation, connectivity is automatically
      | determined, based on the active variant and port name matching.
  In1 : Inport
  Simulation Subsystem : Subsystem  TreatAsAtomicUnit=on  VariantControl=TARGET_CODE_GEN == 0
  Target Code Gen Subsystem : Subsystem  TreatAsAtomicUnit=on  VariantControl="TARGET_CODE_GEN  == 1"
  Out1 : Outport

== system Target_Control_System/Target_Control_System/MainLoop/propMotor_mainLoop/motorTaskMainFastStep(&oProp)/Observer Confidence - Prop/IIR ==
  In : Inport
  1-K : Inport  Port=2
  K : Inport  Port=3
  Product : Product  OutDataTypeStr=single  RndMeth=Zero
  Product1 : Product  RndMeth=Zero
  Sum : Sum  Inputs=|++  OutDataTypeStr=single
  Unit Delay : UnitDelay  SampleTime=-1  HasFrameUpgradeWarning=on
  Out : Outport
  wires:
  Sum/1 -> Unit Delay/1, Out/1
  Unit Delay/1 -> Product/1
  K/1 -> Product1/2
  1-K/1 -> Product/2
  Product/1 -> Sum/1
  Product1/1 -> Sum/2
  In/1 -> Product1/1

== system Target_Control_System/Target_Control_System/MainLoop/propMotor_mainLoop/motorTaskMainFastStep(&oProp)/PWM for Simulation/Subsystem ==
  Enable : EnablePort
  Bus Creator1 : BusCreator  Inputs=3
  Data Store Read7 : DataStoreRead  DataStoreName=oProp  DataStoreElements=oProp.oIsr_.oOut_.uiPwmDutyTicksA_  IndexOptions=Index vector (dialog)  Indices=1  OutputSizes=1
  Data Store Read8 : DataStoreRead  DataStoreName=oProp  DataStoreElements=oProp.oIsr_.oOut_.uiPwmDutyTicksB_  IndexOptions=Index vector (dialog)  Indices=1  OutputSizes=1
  Data Store Read9 : DataStoreRead  DataStoreName=oProp  DataStoreElements=oProp.oIsr_.oOut_.uiPwmDutyTicksC_  IndexOptions=Index vector (dialog)  Indices=1  OutputSizes=1
  propMotor_PWMticks : Outport
  wires:
  Data Store Read8/1 -> Bus Creator1/2  "Bticks"
  Bus Creator1/1 -> propMotor_PWMticks/1
  Data Store Read9/1 -> Bus Creator1/3  "Cticks"
  Data Store Read7/1 -> Bus Creator1/1  "Aticks"

== system Target_Control_System/Target_Control_System/MainLoop/propMotor_mainLoop/motorTaskMainFastStep(&oProp)/PWM for Simulation/Subsystem1 ==
  Enable : EnablePort
  Data Store Read6 : DataStoreRead  DataStoreName=oProp  DataStoreElements=oProp.oMot_.oOut_.uiPwmRequestFromMain_  IndexOptions=Index vector (dialog)  Indices=1  OutputSizes=1
  Scope : Scope
  Subsystem : Subsystem
  propMotor_PWMticks : Outport
  wires:
  Data Store Read6/1 -> Subsystem/Enable, Scope/1
  Subsystem/1(propMotor_PWMticks) -> propMotor_PWMticks/1

== system Target_Control_System/Target_Control_System/MainLoop/pumpMotor_mainLoop/Decimation gate A for 200 Hz Pump/Current offset nulling/initiateOffsetNulling(&oPump) ==
  note: Further checks for starting the nulling process are handled inside the lower level function
  Enable : EnablePort
  Chart : Stateflow chart  TreatAsAtomicUnit=on

== system Target_Control_System/Target_Control_System/MainLoop/pumpMotor_mainLoop/Decimation gate A for 200 Hz Pump/Subsystem/Subsystem ==
  Enable : EnablePort
  Data Store Write1 : DataStoreWrite  DataStoreName=oPump  DataStoreElements=oPump.oMot_.oState_.fIdleCtrlCurrent_  IndexOptions=Index vector (dialog)  Indices=1  OutputSizes=1
  Data Store Write3 : DataStoreWrite  DataStoreName=oPump  DataStoreElements=oPump.oMot_.oParam_.oPiDataIdleCtrl_.fState_  IndexOptions=Index vector (dialog)  Indices=1  OutputSizes=1
  Zero1 : Constant  Value=0  OutDataTypeStr=single  SampleTime=-1
  wires:
  Zero1/1 -> Data Store Write1/1, Data Store Write3/1

== system Target_Control_System/Target_Control_System/MainLoop/pumpMotor_mainLoop/Decimation gate A for 200 Hz Pump/Subsystem/piControllerStep_Idle_Controller ==
  fActual : Inport
  fTarget : Inport  Port=2
  fKp : Inport  Port=3
  fKi : Inport  Port=4
  fScale : Inport  Port=5
  fLoopDt : Inport  Port=6
  fIntMax : Inport  Port=7
  fOutMax : Inport  Port=8
  fIntMin : Inport  Port=9
  fOutMin : Inport  Port=10
  fState : Inport  Port=11
  Enable : EnablePort
  Add : Sum  Inputs=|++
  Data Store Write11 : DataStoreWrite  DataStoreName=oPump  DataStoreElements=oPump.oMot_.oState_.fIdleCtrlCurrent_  IndexOptions=Index vector (dialog)  Indices=1  OutputSizes=1
  Data Store Write2 : DataStoreWrite  DataStoreName=oPump  DataStoreElements=oPump.oMot_.oParam_.oPiDataIdleCtrl_.fState_  IndexOptions=Index vector (dialog)  Indices=1  OutputSizes=1
  Mux : Mux  Inputs=3
  Mux1 : Mux  Inputs=3
  Product : Product
  Saturation Dynamic : simulink/Discontinuities/Saturation Dynamic  OutMin=[]  OutMax=[]  OutDataTypeStr=Inherit: Same as second input  OutDataType=fixdt(1, 16)  OutScaling=2^-10  DoSatur=off
  Saturation Dynamic1 : simulink/Discontinuities/Saturation Dynamic  OutMin=[]  OutMax=[]  OutDataTypeStr=Inherit: Same as second input  OutDataType=fixdt(1, 16)  OutScaling=2^-10  DoSatur=off
  Scope3 : Scope  NumInputPorts=6
  Sum1 : Sum  Inputs=++|
  Sum22 : Sum  Inputs=-+|
  fError * fKi_ * fScale : Fcn  Expr=u(1)*u(2)*u(3)
  fError * fKp_ * fScale1 : Fcn  Expr=u(1)*u(2)*u(3)
  wires:
  Saturation Dynamic1/1 -> Scope3/6, Data Store Write11/1  "fIdleCtrlCurrent_"
  fLoopDt/1 -> Product/2
  fOutMax/1 -> Saturation Dynamic1/1
  fOutMin/1 -> Saturation Dynamic1/3
  fIntMin/1 -> Saturation Dynamic/3
  fIntMax/1 -> Saturation Dynamic/1
  Add/1 -> Saturation Dynamic/2
  fState/1 -> Add/2
  Product/1 -> Add/1
  Mux1/1 -> fError * fKp_ * fScale1/1
  fKi/1 -> Mux/2
  fScale/1 -> Mux/1, Mux1/3
  fKp/1 -> Mux1/2
  Mux/1 -> fError * fKi_ * fScale/1
  Sum1/1 -> Saturation Dynamic1/2  "fError"
  fError * fKp_ * fScale1/1 -> Sum1/1, Scope3/4
  Saturation Dynamic/1 -> Scope3/5, Data Store Write2/1, Sum1/2  "*fpState"
  fActual/1 -> Sum22/1, Scope3/2
  fTarget/1 -> Sum22/2, Scope3/1
  fError * fKi_ * fScale/1 -> Product/1
  Sum22/1 -> Scope3/3, Mux/3, Mux1/1  "fError"

== system Target_Control_System/Target_Control_System/MainLoop/pumpMotor_mainLoop/Decimation gate for 5000 Hz Pump/motorTaskProcessExternalSetpoints(&oPump)/Subsystem1 ==
  passive_holding_mode : TriggerPort  TriggerType=function-call  VariantControl=Variant
  AND5 : Logic  Operator=OR  Inputs=3  AllPortsSameDT=off  OutDataTypeStr=boolean
  Data Store Read85 : DataStoreRead  DataStoreName=oPump  DataStoreElements=oPump.oMot_.oState_.uiDriveState_  IndexOptions=Index vector (dialog)  Indices=1  OutputSizes=1
  Equal1 : RelationalOperator  Operator===  OutDataTypeStr=boolean  RndMeth=Simplest
  Equal13 : RelationalOperator  Operator===  OutDataTypeStr=boolean  RndMeth=Simplest
  Equal2 : RelationalOperator  Operator===  OutDataTypeStr=boolean  RndMeth=Simplest
  Subsystem : Subsystem
  const1 : Constant  Value=226  OutDataTypeStr=uint32  SampleTime=-1
  const2 : Constant  Value=227  OutDataTypeStr=uint32  SampleTime=-1
  const3 : Constant  Value=228  OutDataTypeStr=uint32  SampleTime=-1
  wires:
  const3/1 -> Equal2/2
  const2/1 -> Equal1/2
  const1/1 -> Equal13/2
  Data Store Read85/1 -> Equal13/1, Equal1/1, Equal2/1
  Equal1/1 -> AND5/2
  Equal2/1 -> AND5/3
  AND5/1 -> Subsystem/Enable
  Equal13/1 -> AND5/1

== system Target_Control_System/Target_Control_System/MainLoop/pumpMotor_mainLoop/Decimation gate for 5000 Hz Pump/motorTaskProcessExternalSetpoints(&oPump)/Subsystem2 ==
  hot_standby : TriggerPort  TriggerType=function-call  VariantControl=Variant
  AND5 : Logic  Operator=OR  AllPortsSameDT=off  OutDataTypeStr=boolean
  Data Store Read85 : DataStoreRead  DataStoreName=oPump  DataStoreElements=oPump.oMot_.oState_.uiDriveState_  IndexOptions=Index vector (dialog)  Indices=1  OutputSizes=1
  Equal1 : RelationalOperator  Operator===  OutDataTypeStr=boolean  RndMeth=Simplest
  Equal13 : RelationalOperator  Operator===  OutDataTypeStr=boolean  RndMeth=Simplest
  Subsystem : Subsystem
  const1 : Constant  Value=235  OutDataTypeStr=uint32  SampleTime=-1
  const2 : Constant  Value=236  OutDataTypeStr=uint32  SampleTime=-1
  wires:
  const2/1 -> Equal1/2
  const1/1 -> Equal13/2
  Data Store Read85/1 -> Equal13/1, Equal1/1
  Equal1/1 -> AND5/2
  AND5/1 -> Subsystem/Enable
  Equal13/1 -> AND5/1

== system Target_Control_System/Target_Control_System/MainLoop/pumpMotor_mainLoop/Decimation gate for 5000 Hz Pump/motorTaskProcessExternalSetpoints(&oPump)/Subsystem3 ==
  note: // Position target
  note: // Speed target
  note: Iq current (that is, torque target)
  note: // Do Id
  note: // (Iq is controlled by the forced angle sequencer)
  note: // Forced angle start regime, ensure that Id is zero
  set_target : TriggerPort  TriggerType=function-call  VariantControl=Variant
  AND1 : Logic  AllPortsSameDT=off  OutDataTypeStr=boolean
  AND5 : Logic  Inputs=3  AllPortsSameDT=off  OutDataTypeStr=boolean
  Data Store Read85 : DataStoreRead  DataStoreName=oPump  DataStoreElements=oPump.oMot_.oState_.uiDriveState_  IndexOptions=Index vector (dialog)  Indices=1  OutputSizes=1
  Equal1 : RelationalOperator  OutDataTypeStr=boolean  RndMeth=Simplest
  Equal13 : RelationalOperator  Operator=~=  OutDataTypeStr=boolean  RndMeth=Simplest
  Equal14 : RelationalOperator  Operator=~=  OutDataTypeStr=boolean  RndMeth=Simplest
  Equal2 : RelationalOperator  Operator=<=  OutDataTypeStr=boolean  RndMeth=Simplest
  NOT : Logic  Operator=NOT  AllPortsSameDT=off  OutDataTypeStr=boolean
  NOT1 : Logic  Operator=NOT  AllPortsSameDT=off  OutDataTypeStr=boolean
  Subsystem : Subsystem
  Subsystem1 : Subsystem
  Subsystem2 : Subsystem
  Subsystem3 : Subsystem
  Subsystem4 : Subsystem
  const1 : Constant  Value=245  OutDataTypeStr=uint32  SampleTime=-1
  const17 : Constant  Value=211  OutDataTypeStr=uint32  SampleTime=-1
  const18 : Constant  Value=212  OutDataTypeStr=uint32  SampleTime=-1
  const2 : Constant  Value=254  OutDataTypeStr=uint32  SampleTime=-1
  wires:
  NOT1/1 -> Subsystem4/Enable
  AND5/1 -> NOT1/1, Subsystem3/Enable, Subsystem/Enable, Subsystem1/Enable, Subsystem2/Enable
  Equal13/1 -> AND5/1
  Equal1/1 -> AND1/1
  const18/1 -> Equal14/2
  Equal2/1 -> AND1/2
  AND1/1 -> NOT/1
  const17/1 -> Equal13/1
  Data Store Read85/1 -> Equal2/1, Equal1/1, Equal14/1, Equal13/2
  const2/1 -> Equal2/2
  NOT/1 -> AND5/3
  const1/1 -> Equal1/2
  Equal14/1 -> AND5/2
